simulink model "FCW"  (R2022b)
settings: Solver=VariableStepAuto  StartTime=0.0  StopTime=10.0  RelTol=1e-3
settings Model: Creator=HP  LastModifiedBy=HP

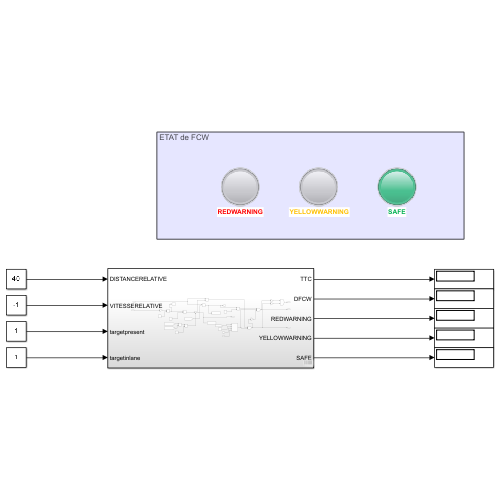
[thumbnail: Simulink's stored preview of the top-level diagram]
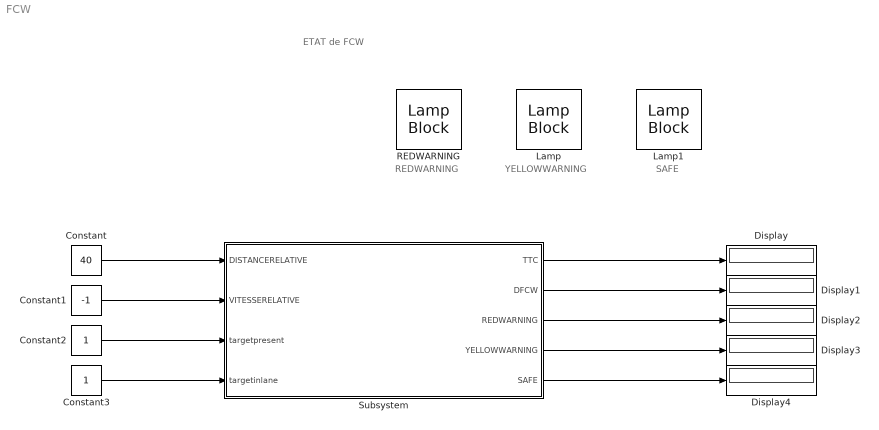
== system FCW ==
  note: ETAT de FCW
  note: SAFE
  note: YELLOWWARNING
  note: REDWARNING
  Constant : Constant  Value=40
  Constant1 : Constant  Value=-1
  Constant2 : Constant
  Constant3 : Constant
  Display{,1..4} (5 alike) : Display
  Lamp : LampBlock  LabelPosition=Hide
  Lamp1 : LampBlock  LabelPosition=Hide
  REDWARNING : LampBlock  LabelPosition=Hide
  Subsystem : Subsystem
  wires:
  Constant/1 -> Subsystem/1(DISTANCERELATIVE)
  Constant1/1 -> Subsystem/2(VITESSERELATIVE)
  Constant2/1 -> Subsystem/3(targetpresent)
  Constant3/1 -> Subsystem/4(targetinlane)
  Subsystem/1(TTC) -> Display/1
  Subsystem/2(DFCW) -> Display1/1
  Subsystem/3(REDWARNING) -> Display2/1
  Subsystem/4(YELLOWWARNING) -> Display3/1
  Subsystem/5(SAFE) -> Display4/1

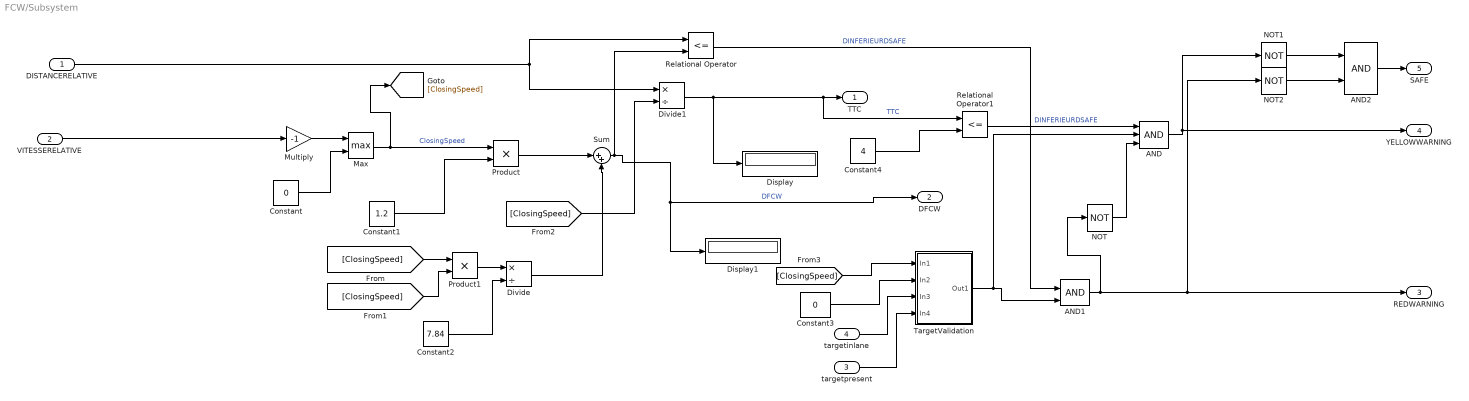
== system FCW/Subsystem ==
  DISTANCERELATIVE : Inport
  VITESSERELATIVE : Inport  Port=2
  targetpresent : Inport  Port=3
  targetinlane : Inport  Port=4
  AND : Logic  Inputs=3  IconShape=distinctive  AllPortsSameDT=off  OutDataTypeStr=boolean
  AND1 : Logic  IconShape=distinctive  AllPortsSameDT=off  OutDataTypeStr=boolean
  AND2 : Logic  IconShape=distinctive  AllPortsSameDT=off  OutDataTypeStr=boolean
  Constant : Constant  Value=0
  Constant1 : Constant  Value=1.2
  Constant2 : Constant  Value=7.84
  Constant3 : Constant  Value=0  VectorParams1D=off  SampleTime=-1
  Constant4 : Constant  Value=4
  Display : Display
  Display1 : Display
  Divide : Product  Inputs=*/
  Divide1 : Product  Inputs=*/
  Max : MinMax  Function=max  Inputs=2
  Multiply : Gain  Gain=-1
  NOT : Logic  Operator=NOT  IconShape=distinctive  AllPortsSameDT=off  OutDataTypeStr=boolean
  NOT1 : Logic  Operator=NOT  IconShape=distinctive  AllPortsSameDT=off  OutDataTypeStr=boolean
  NOT2 : Logic  Operator=NOT  IconShape=distinctive  AllPortsSameDT=off  OutDataTypeStr=boolean
  Product : Product
  Product1 : Product
  Relational Operator : RelationalOperator  Operator=<=  OutDataTypeStr=boolean  RndMeth=Simplest  InputSameDT=off
  Relational Operator1 : RelationalOperator  Operator=<=  OutDataTypeStr=boolean  RndMeth=Simplest  InputSameDT=off
  Sum : Sum  Inputs=|++
  TargetValidation : Subsystem
  TTC : Outport
  DFCW : Outport  Port=2
  REDWARNING : Outport  Port=3
  YELLOWWARNING : Outport  Port=4
  SAFE : Outport  Port=5
  wires:
  VITESSERELATIVE/1 -> Multiply/1
  Constant/1 -> Max/2
  Multiply/1 -> Max/1
  Max/1 -> [ClosingSpeed], Product/1  "ClosingSpeed"
  Constant1/1 -> Product/2
  Product/1 -> Sum/1
  [ClosingSpeed] -> Product1/1
  [ClosingSpeed] -> Product1/2
  Product1/1 -> Divide/1
  Constant2/1 -> Divide/2
  Divide/1 -> Sum/2
  [ClosingSpeed] -> Divide1/2
  Divide1/1 -> Relational Operator1/1, TTC/1, Display/1  "TTC"
  DISTANCERELATIVE/1 -> Relational Operator/1, Divide1/1
  Sum/1 -> Relational Operator/2, DFCW/1, Display1/1  "DFCW"
  Relational Operator/1 -> AND1/1  "DINFERIEURDSAFE"
  [ClosingSpeed] -> TargetValidation/1(In1)
  Constant3/1 -> TargetValidation/2(In2)
  targetinlane/1 -> TargetValidation/3(In3)
  targetpresent/1 -> TargetValidation/4(In4)
  TargetValidation/1(Out1) -> AND/2, AND1/2
  AND1/1 -> NOT/1, NOT2/1, REDWARNING/1
  Constant4/1 -> Relational Operator1/2
  Relational Operator1/1 -> AND/1  "DINFERIEURDSAFE"
  NOT/1 -> AND/3
  AND/1 -> NOT1/1, YELLOWWARNING/1
  NOT1/1 -> AND2/1
  NOT2/1 -> AND2/2
  AND2/1 -> SAFE/1

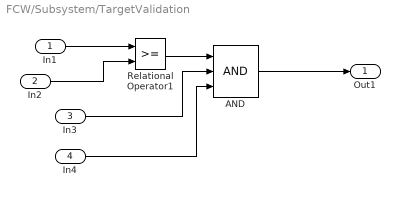
== system FCW/Subsystem/TargetValidation ==
  In1 : Inport
  In2 : Inport  Port=2
  In3 : Inport  Port=3
  In4 : Inport  Port=4
  AND : Logic  Inputs=3  IconShape=distinctive  AllPortsSameDT=off  OutDataTypeStr=boolean
  Relational Operator1 : RelationalOperator  OutDataTypeStr=boolean  RndMeth=Simplest  InputSameDT=off
  Out1 : Outport
  wires:
  In3/1 -> AND/2
  AND/1 -> Out1/1
  Relational Operator1/1 -> AND/1
  In1/1 -> Relational Operator1/1
  In2/1 -> Relational Operator1/2
  In4/1 -> AND/3
